simulink model "power_dcvoltage"  (Simulink 6.0)
settings: Solver=ode23s  SolverMode=SingleTasking  StartTime=0.0  StopTime=0.01  RelTol=1e-3  AbsTol=1e-6
libraries: powerlib x8
settings Model: Creator=patrice  LastModifiedBy=batserve  ExtModeTrigMode=oneshot  ExtModeArmWhenConnect=off  ExtModeAutoUpdateStatusClock=off
settings DataIOCC: LimitDataPoints=off  SignalLoggingName=sigsOut
settings OptimizationCC: BooleanDataType=off
settings DebuggingCC: SolverPrmCheckMsg=none
settings HardwareCC: TargetUnknown=on
settings RTWCC: TemplateMakefile=grt_unix.tmf

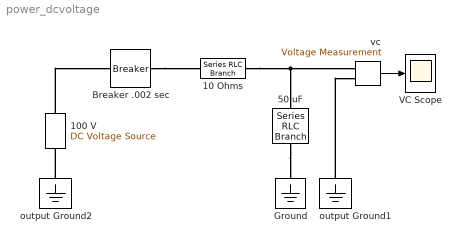
== system power_dcvoltage ==
  10 Ohms : powerlib/Elements/Series RLC Branch  PhysicalDomain=powersysdomain  SubClassName=unknown  LeftPortType=p1  RightPortType=p1  LConnTagsString=__new0  RConnTagsString=__new0  Resistance=10  Inductance=0  Capacitance=inf  Measurements=None
  100 V : powerlib/Electrical Sources/DC Voltage Source  Description=source block  Orientation=up  Amplitude=100  Measurements=None
      settings: AttributesFormatString=\n
  50 uF : powerlib/Elements/Series RLC Branch  Orientation=down  PhysicalDomain=powersysdomain  SubClassName=unknown  LeftPortType=p1  RightPortType=p1  LConnTagsString=__new0  RConnTagsString=__new0  Resistance=0  Inductance=0  Capacitance=50e-6  Measurements=None
  Breaker .002 sec : powerlib/Elements/Breaker  BreakerResistance=0.01  InitialState=0  SnubberResistance=inf  SnubberCapacitance=0  SwitchingTimes=[ .002 ]  External=off  Measurements=None
      settings: AttributesFormatString=\n
  Ground : powerlib/Elements/Ground  Orientation=down  PhysicalDomain=powersysdomain  SubClassName=unknown  LeftPortType=p1  RightPortType=p1  LConnTagsString=a
  VC Scope : Scope
      settings: TickLabels=on  TimeRange=0.01  YMin=-10  YMax=120  DataFormat=Array
  output Ground1 : powerlib/Elements/Ground  Orientation=down  PhysicalDomain=powersysdomain  SubClassName=unknown  LeftPortType=p1  RightPortType=p1  LConnTagsString=a
  output Ground2 : powerlib/Elements/Ground  Orientation=down  PhysicalDomain=powersysdomain  SubClassName=unknown  LeftPortType=p1  RightPortType=p1  LConnTagsString=a
  vc : powerlib/Measurements/Voltage Measurement  Tag=PoWeRsYsTeMmEaSuReMeNt  PhasorSimulation=off  OutputType=Magnitude  PSBequivalent=0
  wires:
  vc/1 -> VC Scope/1
  connections:
  100 V/RConn1 -- Breaker .002 sec/LConn1
  Breaker .002 sec/RConn1 -- 10 Ohms/LConn1
  output Ground2/LConn1 -- 100 V/LConn1
  10 Ohms/RConn1 -- vc/LConn1 -- 50 uF/LConn1
  50 uF/RConn1 -- Ground/LConn1
  output Ground1/LConn1 -- vc/LConn2
